simulink model "CO_120325_Cascaded_Water_Tanks_Simulink"  (R2023b)
settings: Solver=VariableStepAuto  StartTime=0.0  StopTime=1200  FixedStep=1  RelTol=1e-3
values from neighbouring files (symbols this model uses):
  a0 = R_pipe2    (= 1701.41579261)    [CO_120325_Cascaded_Water_Tanks.m]
  b0 = 1    [CO_120325_Cascaded_Water_Tanks.m]
  b1 = A_tank1*R_pipe1 + A_tank2*R_pipe2    (= 1503.32494353)    [CO_120325_Cascaded_Water_Tanks.m]
  b2 = A_tank1*A_tank2*R_pipe1*R_pipe2    (= 564996.47146)    [CO_120325_Cascaded_Water_Tanks.m]
  q_in = 3.4e-3    (= 0.0034)    [CO_120325_Cascaded_Water_Tanks.m]
libraries: slpidlib x1, simulink x1
settings Model: Creator=const  LastModifiedBy=const

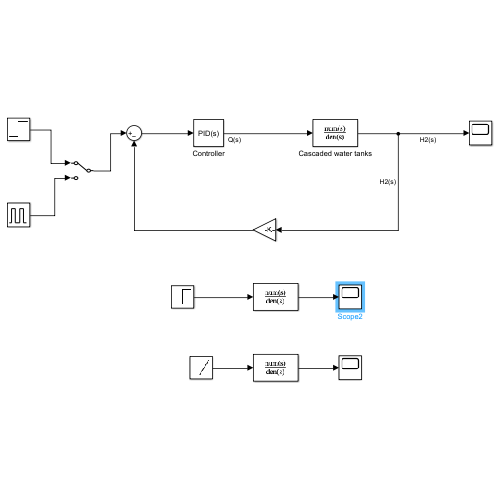
[thumbnail: Simulink's stored preview of the top-level diagram]
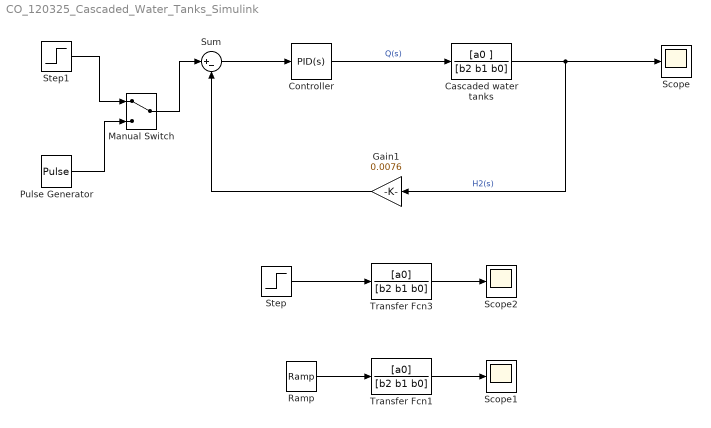
== system CO_120325_Cascaded_Water_Tanks_Simulink ==
  Cascaded water tanks : TransferFcn  Numerator=[a0 ]  Denominator=[b2 b1 b0]
  Controller : slpidlib/PID Controller  Controller=PID  Form=Parallel  TimeDomain=Continuous-time  UseExternalTs=off  SampleTime=-1  IntegratorMethod=Forward Euler  FilterMethod=Forward Euler  ControllerParametersSource=internal  P=3.92/2.6  I=1.23e-3  UseKiTs=off  D=6.265e2  N=100  UseFilter=on  TunerSelectOption=Transfer Function Based (PID Tuner App)  InitialConditionSource=internal  InitialConditionForIntegrator=0  InitialConditionForFilter=0  DifferentiatorICPrevScaledInput=0  ExternalReset=none  TrackingMode=off  Kt=1  LimitOutput=off  SatLimitsSource=internal  UpperSaturationLimit=inf  LowerSaturationLimit=-inf  LinearizeAsGain=on  AntiWindupMode=none  Kb=1  LimitIntegrator=off  UpperIntegratorSaturationLimit=inf  LowerIntegratorSaturationLimit=-inf  POutMin=[]  POutMax=[]  IOutMin=[]  IOutMax=[]  DOutMin=[]  DOutMax=[]  NOutMin=[]  NOutMax=[]  SumOutMin=[]  SumOutMax=[]  SaturationOutMin=[]  SaturationOutMax=[]  PParamMin=[]  PParamMax=[]  IParamMin=[]  IParamMax=[]  DParamMin=[]  DParamMax=[]  NParamMin=[]  NParamMax=[]  KbParamMin=[]  KbParamMax=[]  KtParamMin=[]  KtParamMax=[]  KbOutMin=[]  KbOutMax=[]  KtOutMin=[]  KtOutMax=[]  IntegratorOutMin=[]  IntegratorOutMax=[]  FilterOutMin=[]  FilterOutMax=[]  SumI1OutMin=[]  SumI1OutMax=[]  SumI2OutMin=[]  SumI2OutMax=[]  SumI3OutMin=[]  SumI3OutMax=[]  SumI4OutMin=[]  SumI4OutMax=[]  SumDOutMin=[]  SumDOutMax=[]  DifferentiatorOutMin=[]  DifferentiatorOutMax=[]  FilterDiffOutCoefMin=[]  FilterDiffOutCoefMax=[]  ReciprocalOutMin=[]  ReciprocalOutMax=[]  SumDenOutMin=[]  SumDenOutMax=[]  SumNumOutMin=[]  SumNumOutMax=[]  DivideOutMin=[]  DivideOutMax=[]  UdiffTsProdOutMin=[]  UdiffTsProdOutMax=[]  NTsProdOutMin=[]  NTsProdOutMax=[]  UintegralTsProdOutMin=[]  UintegralTsProdOutMax=[]  UngainTsProdOutMin=[]  UngainTsProdOutMax=[]  ClampingZeroOutDataTypeStr=Inherit: Inherit via back propagation  ClampingZeroOutMin=[]  ClampingZeroOutMax=[]  FilterDenConstantOutDataTypeStr=Inherit: Inherit via back propagation  FilterDenConstantOutMin=[]  FilterDenConstantOutMax=[]  PCopyOutDataTypeStr=Inherit: Inherit via back propagation  PCopyOutMin=[]  PCopyOutMax=[]  NCopyOutDataTypeStr=Inherit: Inherit via back propagation  NCopyOutMin=[]  NCopyOutMax=[]  IntegratorContinuousStateAttributes=''  IntegratorStateMustResolveToSignalObject=off  IntegratorRTWStateStorageClass=Auto  FilterContinuousStateAttributes=''  FilterStateMustResolveToSignalObject=off  FilterRTWStateStorageClass=Auto  ParallelPVariant=InternalParameters  IdealPVariant=Disabled  IVariant=InternalParameters  DVariant=InternalParameters  IntegratorVariant=Continuous  SatVariant=Disabled  AWVariant=Passthrough  PCopyVariant=Disabled  TRVariant=Disabled  FdbkBlocksVariant=Forward  IdealPFdbkVariant=Disabled  SatFdbkVariant=Disabled  DerivativeFilterVariant=ContFilter  NVariant=InternalParameters  NCopyVariant=Disabled  FilterICVariant=InternalICsFilter  IntegratorICVariant=InternalICs  ExternalResetVariant=Disabled  TRSumVariant=Passthrough  SumFdbkVariant=Disabled  SumVariant=Sum_PID  TsampFilterVariant=InternalTs  TsampNgainVariant=Passthrough  TsampIntegralVariant=Disabled_SignalSpec  ExternalSaturationOutDataTypeStr=Inherit: Same as second input
  Gain1 : Gain  Gain=0.0076
  Manual Switch : ManualSwitch
  Pulse Generator : DiscretePulseGenerator  PulseType=Time based  Amplitude=q_in  Period=1200  PulseWidth=50
  Ramp : simulink/Sources/Ramp  slope=q_in  start=0  InitialOutput=0
  Scope : Scope
  Scope1 : Scope
  Scope2 : Scope
  Step : Step  Time=0  After=q_in  SampleTime=0
  Step1 : Step  Time=0  After=q_in  SampleTime=0
  Sum : Sum  Inputs=|+-
  Transfer Fcn1 : TransferFcn  Numerator=[a0]  Denominator=[b2 b1 b0]
  Transfer Fcn3 : TransferFcn  Numerator=[a0]  Denominator=[b2 b1 b0]
  wires:
  Cascaded water tanks/1 -> Gain1/1, Scope/1  "H2(s)"
  Step/1 -> Transfer Fcn3/1
  Transfer Fcn3/1 -> Scope2/1
  Transfer Fcn1/1 -> Scope1/1
  Ramp/1 -> Transfer Fcn1/1
  Manual Switch/1 -> Sum/1
  Step1/1 -> Manual Switch/1
  Pulse Generator/1 -> Manual Switch/2
  Controller/1 -> Cascaded water tanks/1  "Q(s)"
  Sum/1 -> Controller/1
  Gain1/1 -> Sum/2
